simulink model "E_nonlinearB"  (R2017a)
settings: Solver=FixedStepAuto  StartTime=0.0  StopTime=200  FixedStep=sim_time  RelTol=1e-3  EnableMultiTasking=on
values from neighbouring files (symbols this model uses):
  B = [1 0.5 -0.5 -1 0 0.5 ; 0 0 0 0 2 0 ; -0.05 -0.02 0.02 0.05 0 2 ; -1 -1 -1 -1 -2 0]    [A_runSimulation.m]    (also in C_runSimulation.m; D_runSimulation.m; E_runSimulation.m; F_runSimulation.m)
  gain_four = rand()*2    [A_runSimulation.m]    (also in C_runSimulation.m = 0; D_runSimulation.m; E_runSimulation.m = 0; F_runSimulation.m = 0)
  gain_one = rand()*2    [A_runSimulation.m]    (also in C_runSimulation.m = 0; D_runSimulation.m; E_runSimulation.m = 0; F_runSimulation.m = 0)
  gain_three = rand()*2    [A_runSimulation.m]    (also in C_runSimulation.m = 0; D_runSimulation.m; E_runSimulation.m = 0; F_runSimulation.m = 0)
  gain_two = rand()*2    [A_runSimulation.m]    (also in C_runSimulation.m = 0; D_runSimulation.m; E_runSimulation.m = 0; F_runSimulation.m = 0)
  nl_gain = j    [E_runSimulation.m]
  Ql = [0 -0.1 0 0 -0.05 0; -0.2 0 0 0 -0.1 0; 0 0 0 0.2 0.1 0; 0 0 0.1 0 0.05 0; 0 0 0 0 0 0; 0 0 0 0 0 0]    [E_runSimulation.m]
  Qm = [0 0 0 0 -0.1 0; 0 0 0 0 -0.2 0; 0 0 0 0 -0.2 0; 0 0 0 0 -0.1 0; 0 0 0 0 0 0; 0 0 0 0 0 0]    [E_runSimulation.m]
  Qn = [0 -0.025 0 0 0 0; -0.05 0 0 0 0 0; 0 0 0 0.05 0 0; 0 0 0 0.025 0 0; 0 0 0 0 0 0; 0 0 0 0 0 0]    [E_runSimulation.m]
  Qz = [0 -0.2 0 0 -0.05 0; -0.2 0 0 0 -0.1 0; 0 0 0 -0.2 -0.1 0; 0 0 -0.2 0 -0.05 0; 0 0 0 0 0 0; 0 0 0 0 0 0]    [E_runSimulation.m]
  seed_four = k + 30    [A_runSimulation.m]    (also in C_runSimulation.m; D_runSimulation.m; E_runSimulation.m; F_runSimulation.m)
  seed_one = k    [A_runSimulation.m]    (also in C_runSimulation.m; D_runSimulation.m; E_runSimulation.m; F_runSimulation.m)
  seed_three = k + 20    [A_runSimulation.m]    (also in C_runSimulation.m; D_runSimulation.m; E_runSimulation.m; F_runSimulation.m)
  seed_two = k + 10    [A_runSimulation.m]    (also in C_runSimulation.m; D_runSimulation.m; E_runSimulation.m; F_runSimulation.m)
  signal_gain = j    [A_runSimulation.m]    (also in C_runSimulation.m; D_runSimulation.m; E_runSimulation.m = 0.3; F_runSimulation.m)
  sim_time = 1    [E_runSimulation.m]    (also in F_runSimulation.m = 0.1; F_runSimulation2.m = 0.1; G_runSimulation.m = 0.001)
  simulate_envelope = 1    [A_runSimulation.m]    (also in C_runSimulation.m = 0; D_runSimulation.m; E_runSimulation.m = 0)
  u_lim = [[-0.5 -0.5 -0.5 -0.5 -0.5 -0.5]' [0.5 0.5 0.5 0.5 0.5 0.5]']    [A_runSimulation.m]    (also in C_runSimulation.m; D_runSimulation.m; E_runSimulation.m; F_runSimulation.m)
  udot_lim = [[2 2 2 2 2 2]']    [A_runSimulation.m]    (also in C_runSimulation.m; D_runSimulation.m; E_runSimulation.m; F_runSimulation.m)
  W = eye(6)    [A_runSimulation.m]    (also in C_runSimulation.m; D_runSimulation.m; E_runSimulation.m; F_runSimulation.m)
libraries: dspsrcs4 x8
settings Model: Creator=markvoskuijl  LastModifiedBy=Luca
settings DataIOCC: LimitDataPoints=on  SaveFormat=Array  SignalLoggingSaveFormat=ModelDataLogs
settings OptimizationCC: ExpressionDepthLimit=2147483647  LifeSpan=inf
settings DebuggingCC: UnderspecifiedInitializationDetection=Classic  MergeDetectMultiDrivingBlocksExec=none  SolverPrmCheckMsg=warning  FcnCallInpInsideContextMsg=warning  StateNameClashWarn=warning  SFUnexpectedBacktrackingDiag=warning  SFNoUnconditionalDefaultTransitionDiag=warning  SFExecutionAtInitializationDiag=none
settings HardwareCC: ProdBitPerPointer=32  ProdBitPerSizeT=32  ProdBitPerPtrDiffT=32  ProdLargestAtomicFloat=None  ProdIntDivRoundTo=Undefined  ProdEndianess=Unspecified  ProdWordSize=32  ProdHWDeviceType=32-bit Generic
settings ModelReferenceCC: PropagateSignalLabelsOutOfModel=off
settings GRTTargetCC: TargetLangStandard=C89/C90 (ANSI)  GeneratePreprocessorConditionals=Disable all  CombineOutputUpdateFcns=off  GRTInterface=on
settings ConfigComp: CovMetricSettings=dw  CovHtmlReporting=on  CovSaveCumulativeToWorkspaceVar=on  CovSaveSingleToWorkspaceVar=on  CovExternalEMLEnable=off

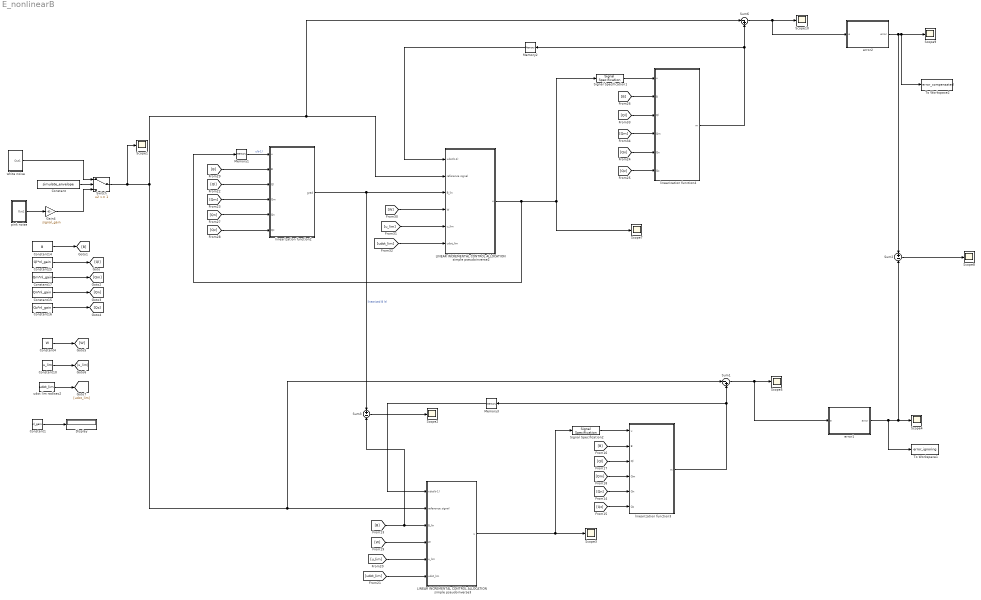
== system E_nonlinearB ==
  Constant : Constant  Value=simulate_envelope
  Constant1 : Constant  Value=nl_gain
  Constant10 : Constant  Value=u_lim
  Constant14 : Constant  Value=B
  Constant15 : Constant  Value=Qn*nl_gain
  Constant16 : Constant  Value=Qz*nl_gain
  Constant17 : Constant  Value=Qm*nl_gain
  Constant25 : Constant  Value=Ql*nl_gain
  Constant4 : Constant  Value=W
  Display : Display
  Gain4 : Gain  Gain=signal_gain
  LINEAR INCREMENTAL CONTROL ALLOCATION simple pseudoinverse2 : Subsystem
  LINEAR INCREMENTAL CONTROL ALLOCATION simple pseudoinverse3 : Subsystem
  Memory1 : Memory  X0=[0 0 0 0 0 0]
  Memory2 : Memory  X0=[0 0 0 0]
  Memory3 : Memory  X0=[0 0 0 0]
  Scope{1..5,7..10} (9 alike) : Scope
  Signal Specification1 : SignalSpecification  Dimensions=[6 1]
  Signal Specification2 : SignalSpecification  Dimensions=[6 1]
  Sum1 : Sum  Inputs=|-+
  Sum2 : Sum  Inputs=+|-
  Sum3 : Sum  Inputs=+|-
  Sum6 : Sum  Inputs=|-+
  Switch : Switch  Threshold=1
  To Workspace1 : ToWorkspace  VariableName=error_ignoring  SampleTime=-1
      settings: Save2DSignal=2-D array (concatenate along first dimension)
  To Workspace2 : ToWorkspace  VariableName=error_compensated  SampleTime=-1
      settings: Save2DSignal=2-D array (concatenate along first dimension)
  error1 : MATLAB Function  TreatAsAtomicUnit=on
  error2 : MATLAB Function  TreatAsAtomicUnit=on
  linearization function2 : MATLAB Function  TreatAsAtomicUnit=on
  linearization function3 : MATLAB Function  TreatAsAtomicUnit=on
  linearization function4 : MATLAB Function  TreatAsAtomicUnit=on
  pink noise : Subsystem
  udot lim rad/sec2 : Constant  Value=udot_lim
  white noise : Subsystem
  wires:
  Constant/1 -> Switch/2
  white noise/1(Out1) -> Switch/1
  Gain4/1 -> Switch/3
  pink noise/1(Out1) -> Gain4/1
  [W] -> LINEAR INCREMENTAL CONTROL ALLOCATION simple pseudoinverse3/4(W)
  [udot_lim] -> LINEAR INCREMENTAL CONTROL ALLOCATION simple pseudoinverse3/6(udot_lim)
  [u_lim] -> LINEAR INCREMENTAL CONTROL ALLOCATION simple pseudoinverse3/5(u_lim)
  LINEAR INCREMENTAL CONTROL ALLOCATION simple pseudoinverse3/1(u) -> Signal Specification2/1, Scope3/1
  Sum1/1 -> error1/1(e), Scope5/1
  Constant14/1 -> [B]
  Constant17/1 -> [Qm]
  Constant15/1 -> [Qn]
  Constant16/1 -> [Qz]
  Constant4/1 -> [W]
  udot lim rad/sec2/1 -> [udot_lim]
  Constant10/1 -> [u_lim]
  [B] -> linearization function3/2(B)
  [Ql] -> linearization function3/3(Ql)
  [Qn] -> linearization function3/5(Qn)
  [Qz] -> linearization function3/6(Qz)
  [Qm] -> linearization function3/4(Qm)
  error1/1(error) -> To Workspace1/1, Sum2/2, Scope4/1
  [Qz] -> linearization function2/6(Qz)
  [Ql] -> linearization function4/3(Ql)
  [B] -> linearization function4/2(B)
  [Qn] -> linearization function4/5(Qn)
  [u_lim] -> LINEAR INCREMENTAL CONTROL ALLOCATION simple pseudoinverse2/5(u_lim)
  Memory1/1 -> linearization function2/1(u)  "u(t-1)"
  Sum6/1 -> error2/1(e), Scope10/1
  linearization function2/1(grad) -> LINEAR INCREMENTAL CONTROL ALLOCATION simple pseudoinverse2/3(B_lin), Sum3/1  "linearized B (t)"
  Sum2/1 -> Scope8/1
  [udot_lim] -> LINEAR INCREMENTAL CONTROL ALLOCATION simple pseudoinverse2/6(udot_lim)
  [Ql] -> linearization function2/3(Ql)
  [W] -> LINEAR INCREMENTAL CONTROL ALLOCATION simple pseudoinverse2/4(W)
  [Qz] -> linearization function4/6(Qz)
  [Qn] -> linearization function2/5(Qn)
  [Qm] -> linearization function2/4(Qm)
  [B] -> linearization function2/2(B)
  [Qm] -> linearization function4/4(Qm)
  Memory2/1 -> LINEAR INCREMENTAL CONTROL ALLOCATION simple pseudoinverse2/1(xdot(t-1))
  Signal Specification1/1 -> linearization function4/1(u)
  Signal Specification2/1 -> linearization function3/1(u)
  Memory3/1 -> LINEAR INCREMENTAL CONTROL ALLOCATION simple pseudoinverse3/1(xdot(t-1))
  linearization function3/1(m) -> Memory3/1, Sum1/2
  Sum3/1 -> Scope2/1
  [B] -> LINEAR INCREMENTAL CONTROL ALLOCATION simple pseudoinverse3/3(B_lin), Sum3/2
  Constant25/1 -> [Ql]
  Switch/1 -> Sum6/1, LINEAR INCREMENTAL CONTROL ALLOCATION simple pseudoinverse2/2(reference signal), LINEAR INCREMENTAL CONTROL ALLOCATION simple pseudoinverse3/2(reference signal), Sum1/1, Scope1/1
  error2/1(error) -> Scope9/1, To Workspace2/1, Sum2/1
  LINEAR INCREMENTAL CONTROL ALLOCATION simple pseudoinverse2/1(u) -> Signal Specification1/1, Scope7/1, Memory1/1
  linearization function4/1(m) -> Memory2/1, Sum6/2
  Constant1/1 -> Display/1

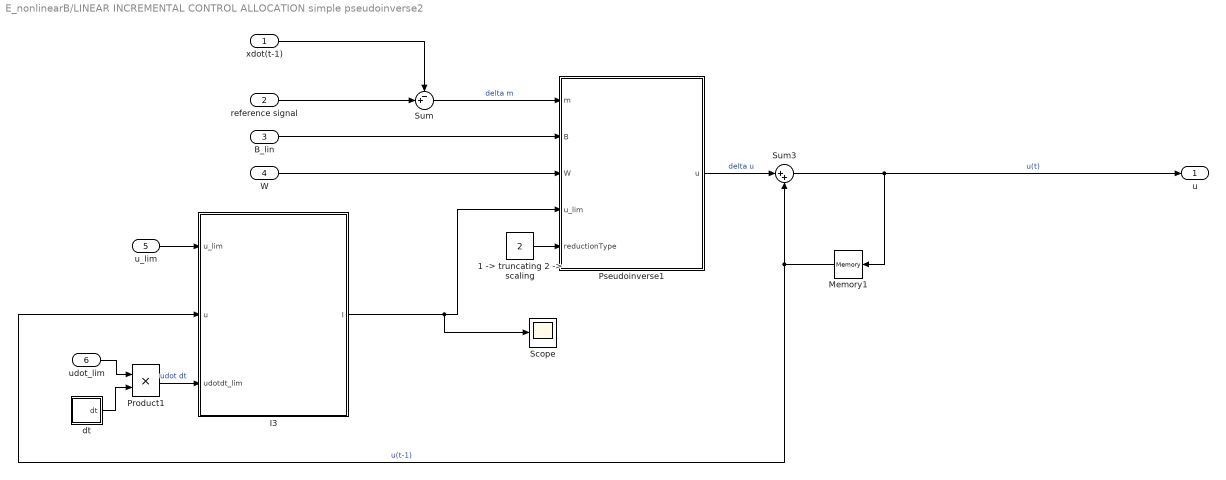
== system E_nonlinearB/LINEAR INCREMENTAL CONTROL ALLOCATION simple pseudoinverse2 ==
  xdot(t-1) : Inport
  reference signal : Inport  Port=2
  B_lin : Inport  Port=3
  W : Inport  Port=4
  u_lim : Inport  Port=5
  udot_lim : Inport  Port=6
  "1 -> truncating 2 -> scaling" : Constant  Value=2
  I3 : MATLAB Function  TreatAsAtomicUnit=on
  Memory1 : Memory
  Product1 : Product
  Pseudoinverse1 : MATLAB Function  TreatAsAtomicUnit=on
  Scope : Scope
  Sum : Sum  Inputs=-+|
  Sum3 : Sum  Inputs=|++
  dt : Subsystem
  u : Outport
  wires:
  reference signal/1 -> Sum/2
  I3/1(I) -> Scope/1, Pseudoinverse1/4(u_lim)
  Memory1/1 -> I3/2(u), Sum3/2  "u(t-1)"
  Product1/1 -> I3/3(udotdt_lim)  "udot dt"
  udot_lim/1 -> Product1/1
  Sum3/1 -> u/1, Memory1/1  "u(t)"
  Pseudoinverse1/1(u) -> Sum3/1  "delta u"
  dt/1(dt) -> Product1/2
  Sum/1 -> Pseudoinverse1/1(m)  "delta m"
  B_lin/1 -> Pseudoinverse1/2(B)
  u_lim/1 -> I3/1(u_lim)
  W/1 -> Pseudoinverse1/3(W)
  "1 -> truncating 2 -> scaling"/1 -> Pseudoinverse1/5(reductionType)
  xdot(t-1)/1 -> Sum/1

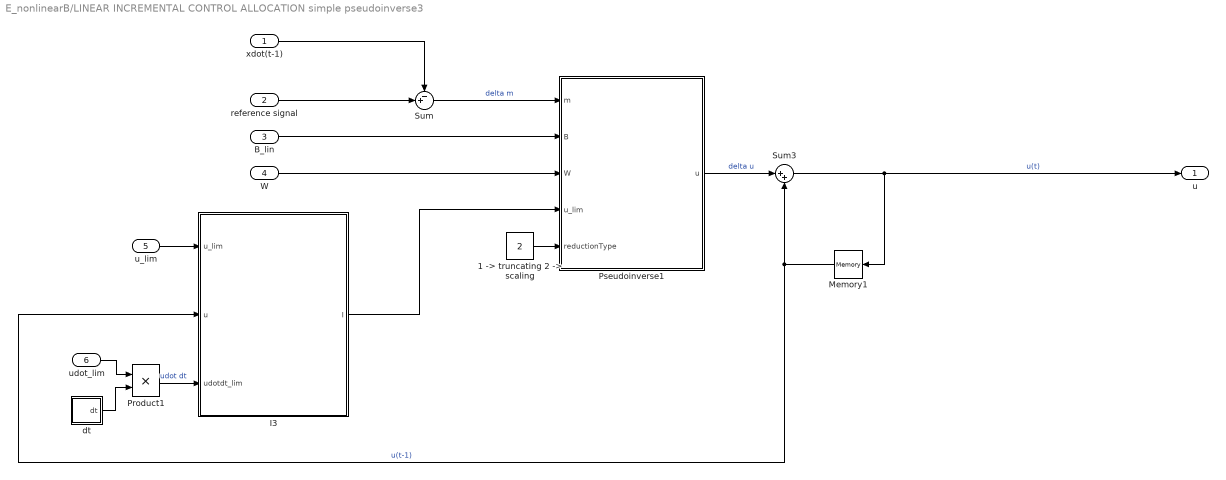
== system E_nonlinearB/LINEAR INCREMENTAL CONTROL ALLOCATION simple pseudoinverse3 ==
  xdot(t-1) : Inport
  reference signal : Inport  Port=2
  B_lin : Inport  Port=3
  W : Inport  Port=4
  u_lim : Inport  Port=5
  udot_lim : Inport  Port=6
  "1 -> truncating 2 -> scaling" : Constant  Value=2
  I3 : MATLAB Function  TreatAsAtomicUnit=on
  Memory1 : Memory
  Product1 : Product
  Pseudoinverse1 : MATLAB Function  TreatAsAtomicUnit=on
  Sum : Sum  Inputs=-+|
  Sum3 : Sum  Inputs=|++
  dt : Subsystem
  u : Outport
  wires:
  reference signal/1 -> Sum/2
  I3/1(I) -> Pseudoinverse1/4(u_lim)
  Memory1/1 -> I3/2(u), Sum3/2  "u(t-1)"
  Product1/1 -> I3/3(udotdt_lim)  "udot dt"
  udot_lim/1 -> Product1/1
  Sum3/1 -> u/1, Memory1/1  "u(t)"
  Pseudoinverse1/1(u) -> Sum3/1  "delta u"
  dt/1(dt) -> Product1/2
  Sum/1 -> Pseudoinverse1/1(m)  "delta m"
  B_lin/1 -> Pseudoinverse1/2(B)
  u_lim/1 -> I3/1(u_lim)
  W/1 -> Pseudoinverse1/3(W)
  "1 -> truncating 2 -> scaling"/1 -> Pseudoinverse1/5(reductionType)
  xdot(t-1)/1 -> Sum/1

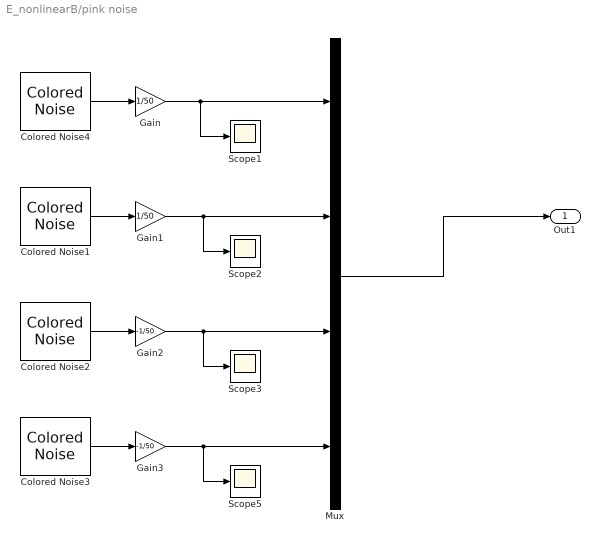
== system E_nonlinearB/pink noise ==
  Colored Noise1 : dspsrcs4/Colored Noise  Color=custom  InverseFrequencyPower=2  NumChannels=1  OutputDataType=single  SamplesPerFrame=1  SampleTime=sim_time  RandomStream=mt19937ar with seed  Seed=seed_two  SimulateUsing=Interpreted execution
      settings: SourceProductName=DSP System Toolbox  SourceProductBaseCode=DS
  Colored Noise2 : dspsrcs4/Colored Noise  Color=custom  InverseFrequencyPower=2  NumChannels=1  OutputDataType=single  SamplesPerFrame=1  SampleTime=sim_time  RandomStream=mt19937ar with seed  Seed=seed_three  SimulateUsing=Interpreted execution
      settings: SourceProductName=DSP System Toolbox  SourceProductBaseCode=DS
  Colored Noise3 : dspsrcs4/Colored Noise  Color=custom  InverseFrequencyPower=2  NumChannels=1  OutputDataType=single  SamplesPerFrame=1  SampleTime=sim_time  RandomStream=mt19937ar with seed  Seed=seed_four  SimulateUsing=Interpreted execution
      settings: SourceProductName=DSP System Toolbox  SourceProductBaseCode=DS
  Colored Noise4 : dspsrcs4/Colored Noise  Color=custom  InverseFrequencyPower=2  NumChannels=1  OutputDataType=single  SamplesPerFrame=1  SampleTime=sim_time  RandomStream=mt19937ar with seed  Seed=seed_one  SimulateUsing=Interpreted execution
      settings: SourceProductName=DSP System Toolbox  SourceProductBaseCode=DS
  Gain : Gain  Gain=1/50
  Gain1 : Gain  Gain=1/50
  Gain2 : Gain  Gain=-1/50
  Gain3 : Gain  Gain=-1/50
  Mux : Mux
  Scope{1..3,5} (4 alike) : Scope
  Out1 : Outport
  wires:
  Colored Noise4/1 -> Gain/1
  Colored Noise1/1 -> Gain1/1
  Colored Noise2/1 -> Gain2/1
  Gain/1 -> Scope1/1, Mux/1
  Gain1/1 -> Scope2/1, Mux/2
  Gain2/1 -> Scope3/1, Mux/3
  Mux/1 -> Out1/1
  Gain3/1 -> Mux/4, Scope5/1
  Colored Noise3/1 -> Gain3/1

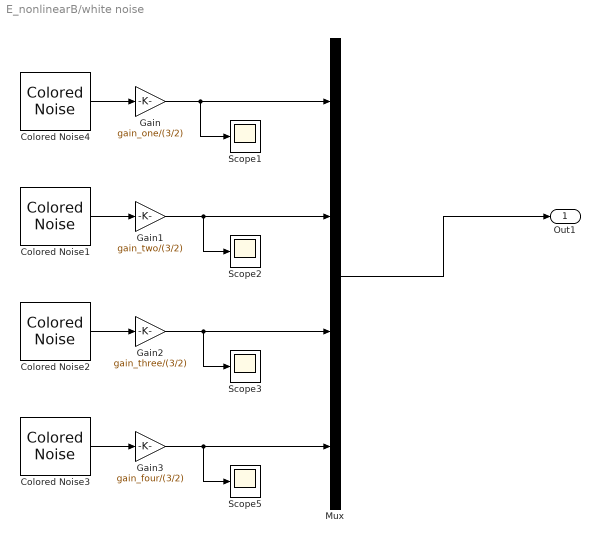
== system E_nonlinearB/white noise ==
  Colored Noise1 : dspsrcs4/Colored Noise  Color=white  InverseFrequencyPower=2  NumChannels=1  OutputDataType=single  SamplesPerFrame=1  SampleTime=sim_time  RandomStream=mt19937ar with seed  Seed=seed_two  SimulateUsing=Interpreted execution
      settings: SourceProductName=DSP System Toolbox  SourceProductBaseCode=DS
  Colored Noise2 : dspsrcs4/Colored Noise  Color=white  InverseFrequencyPower=2  NumChannels=1  OutputDataType=single  SamplesPerFrame=1  SampleTime=sim_time  RandomStream=mt19937ar with seed  Seed=seed_three  SimulateUsing=Interpreted execution
      settings: SourceProductName=DSP System Toolbox  SourceProductBaseCode=DS
  Colored Noise3 : dspsrcs4/Colored Noise  Color=white  InverseFrequencyPower=2  NumChannels=1  OutputDataType=single  SamplesPerFrame=1  SampleTime=sim_time  RandomStream=mt19937ar with seed  Seed=seed_four  SimulateUsing=Interpreted execution
      settings: SourceProductName=DSP System Toolbox  SourceProductBaseCode=DS
  Colored Noise4 : dspsrcs4/Colored Noise  Color=white  InverseFrequencyPower=2  NumChannels=1  OutputDataType=single  SamplesPerFrame=1  SampleTime=sim_time  RandomStream=mt19937ar with seed  Seed=seed_one  SimulateUsing=Interpreted execution
      settings: SourceProductName=DSP System Toolbox  SourceProductBaseCode=DS
  Gain : Gain  Gain=gain_one/(3/2)
  Gain1 : Gain  Gain=gain_two/(3/2)
  Gain2 : Gain  Gain=gain_three/(3/2)
  Gain3 : Gain  Gain=gain_four/(3/2)
  Mux : Mux
  Scope{1..3,5} (4 alike) : Scope
  Out1 : Outport
  wires:
  Colored Noise4/1 -> Gain/1
  Colored Noise1/1 -> Gain1/1
  Colored Noise2/1 -> Gain2/1
  Gain/1 -> Scope1/1, Mux/1
  Gain1/1 -> Scope2/1, Mux/2
  Gain2/1 -> Scope3/1, Mux/3
  Mux/1 -> Out1/1
  Gain3/1 -> Mux/4, Scope5/1
  Colored Noise3/1 -> Gain3/1

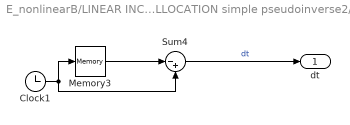
== system E_nonlinearB/LINEAR INCREMENTAL CONTROL ALLOCATION simple pseudoinverse2/dt ==
  Clock1 : Clock
  Memory3 : Memory
  Sum4 : Sum  Inputs=|-+
  dt : Outport
  wires:
  Clock1/1 -> Sum4/2, Memory3/1
  Memory3/1 -> Sum4/1
  Sum4/1 -> dt/1  "dt"

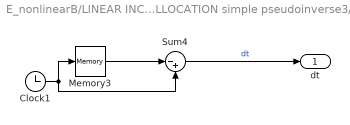
== system E_nonlinearB/LINEAR INCREMENTAL CONTROL ALLOCATION simple pseudoinverse3/dt ==
  Clock1 : Clock
  Memory3 : Memory
  Sum4 : Sum  Inputs=|-+
  dt : Outport
  wires:
  Clock1/1 -> Sum4/2, Memory3/1
  Memory3/1 -> Sum4/1
  Sum4/1 -> dt/1  "dt"

== matlab function E_nonlinearB/LINEAR INCREMENTAL CONTROL ALLOCATION simple pseudoinverse2/I3 ==
  data: u_lim input; u input; udotdt_lim input; I output
function I = computeIntersection(u_lim, u, udotdt_lim)
%check if the matrices are correct
    if not(isequal(size(u_lim,1),size(udotdt_lim,1), size(u,1)))
        error ('input matrix dimensions do not match')
    end

%declare space of intersection
    I = zeros(length(u_lim),2);
    
    I(:,1) = -min(udotdt_lim, abs(u_lim(:,1)-u));
    I(:,2) = min(+udotdt_lim, abs(u_lim(:,2)-u));
    
end

== matlab function E_nonlinearB/LINEAR INCREMENTAL CONTROL ALLOCATION simple pseudoinverse3/Pseudoinverse1 ==
  data: m input; u output; B input; W input; u_lim input; reductionType input
function u = Pseudoinverse(m, B, W, u_lim, reductionType)
coder.varsize('u_index', 'Br', 'Wr', 'u_sat');

%check if the matrices are correct
    if not(isequal(size(u_lim,1),size(B,2),size(W,1),size(W,2))...
       && isequal(length(m),size(B,1)))
        error ('input matrix dimensions do not match')
    end
    
%assign to every equation an index    
    u_index = [1:length(u_lim)].';
    
%check the type of system and then compute the pseudoinverse 1st step
    order = size(B,2)-size(B,1);

    if order > 0 %over-determined, solution that minimizes the 2norm
        u = inv(W)*B'*inv(B*inv(W)*B')*m;
    elseif order < 0 %under-determined, solution that minimizes the error
        u = inv(B'*B)*B'*m;   
    else %order = 0, sqared thus invertiBrle
        u = inv(B)*m;
    end

%deifne u_sat vector
    u_sat = zeros(length(u),1);
    
%check if the first iteration solution is correct then return    
    if not(any(u < u_lim(:,1))||any(u > u_lim(:,2)))  
        return
    end
    
%The software continues only if the solution has to be reduced
%reduce their value
    switch reductionType
        case 1 %truncation
            %takes note of which one are out of their bounds
                u_sat(u < u_lim(:,1)) = 1;
                u_sat(u > u_lim(:,2)) = 1;
                
            %trucate
                u = min(u, u_lim(:,2));
                u = max(u, u_lim(:,1));

        case 2 %scaling solution -> direction preserving
            %reduce
                a = zeros(length(u),1);

                for i = 1:length(u)
                    if u(i)>0
                       a(i) = abs(u(i)/u_lim(i,2));
                    elseif u(i)<0
                       a(i) = abs(u(i)/u_lim(i,1));
                    else
                       a(i) = 0; 
                    end          
                end
                a_max = max(a);
                u = u/a_max;
            
            %takes note of which one are out of their bounds
                u_sat(u == u_lim(:,2)) = 1;
                u_sat(u == u_lim(:,1)) = 1;
            
    end
    
return
    
end

== matlab function E_nonlinearB/LINEAR INCREMENTAL CONTROL ALLOCATION simple pseudoinverse3/I3 ==
  data: u_lim input; u input; udotdt_lim input; I output
function I = computeIntersection(u_lim, u, udotdt_lim)
%check if the matrices are correct
    if not(isequal(size(u_lim,1),size(udotdt_lim,1), size(u,1)))
        error ('input matrix dimensions do not match')
    end

%declare space of intersection
    I = zeros(length(u_lim),2);
    
    I(:,1) = -min(udotdt_lim, abs(u_lim(:,1)-u));
    I(:,2) = min(+udotdt_lim, abs(u_lim(:,2)-u));
    
end

== matlab function E_nonlinearB/linearization function3 ==
  data: u input; B input; m output; Ql input; Qm input; Qn input; Qz input
function m = moment(u, B, Ql, Qm, Qn, Qz)
%the equation here implemented comes from the article
%"A method fot including control effector interactions in the control
%allocation problem" by Oppenheimer but it is addressed to control also z
%The equation is posed in te form:

%             |u' Ql|
%             |u' Qm|
%   g = 1/2 * |u' Qn| + B
%             |u' Qz|

m = ((1/2)*([u.'*Ql; u.'*Qm; u.'*Qn; u.'*Qz])+B)*u;

end

== matlab function E_nonlinearB/error1 ==
  data: e input; error output
function error = error(e)

    error = sum(abs(e));

end

== matlab function E_nonlinearB/LINEAR INCREMENTAL CONTROL ALLOCATION simple pseudoinverse2/Pseudoinverse1 ==
  data: m input; u output; B input; W input; u_lim input; reductionType input
function u = Pseudoinverse(m, B, W, u_lim, reductionType)
coder.varsize('u_index', 'Br', 'Wr', 'u_sat');

%check if the matrices are correct
    if not(isequal(size(u_lim,1),size(B,2),size(W,1),size(W,2))...
       && isequal(length(m),size(B,1)))
        error ('input matrix dimensions do not match')
    end
    
%assign to every equation an index    
    u_index = [1:length(u_lim)].';
    
%check the type of system and then compute the pseudoinverse 1st step
    order = size(B,2)-size(B,1);

    if order > 0 %over-determined, solution that minimizes the 2norm
        u = inv(W)*B'*inv(B*inv(W)*B')*m;
    elseif order < 0 %under-determined, solution that minimizes the error
        u = inv(B'*B)*B'*m;   
    else %order = 0, sqared thus invertiBrle
        u = inv(B)*m;
    end

%deifne u_sat vector
    u_sat = zeros(length(u),1);
    
%check if the first iteration solution is correct then return    
    if not(any(u < u_lim(:,1))||any(u > u_lim(:,2)))  
        return
    end
    
%The software continues only if the solution has to be reduced
%reduce their value
    switch reductionType
        case 1 %truncation
            %takes note of which one are out of their bounds
                u_sat(u < u_lim(:,1)) = 1;
                u_sat(u > u_lim(:,2)) = 1;
                
            %trucate
                u = min(u, u_lim(:,2));
                u = max(u, u_lim(:,1));

        case 2 %scaling solution -> direction preserving
            %reduce
                a = zeros(length(u),1);

                for i = 1:length(u)
                    if u(i)>0
                       a(i) = abs(u(i)/u_lim(i,2));
                    elseif u(i)<0
                       a(i) = abs(u(i)/u_lim(i,1));
                    else
                       a(i) = 0; 
                    end          
                end
                a_max = max(a);
                u = u/a_max;
            
            %takes note of which one are out of their bounds
                u_sat(u == u_lim(:,2)) = 1;
                u_sat(u == u_lim(:,1)) = 1;
            
    end
    
    u = real(u);
return
    
end

== matlab function E_nonlinearB/error2 ==
  data: e input; error output
function error = error(e)

    error = sum(abs(e));

end

== matlab function E_nonlinearB/linearization function2 ==
  data: u input; B input; grad output; Ql input; Qm input; Qn input; Qz input
function grad = linearizeSystem(u, B, Ql, Qm, Qn, Qz)
%the equation here implemented comes from the article
%"A method fot including control effector interactions in the control
%allocation problem" by Oppenheimer but it is addressed to control also z
%The equation is posed in te form:

%             |u' Ql|
%             |u' Qm|
%   g = 1/2 * |u' Qn| + B
%             |u' Qz|

%and must be linearized into a new control effectiveness matrix



%check the magnitude of numbers inside the matrices
%     oom = [min(floor(log10(u+1))), min(min(floor(log10(Ql+1)))),...
%         min(min(floor(log10(Qm+1)))), min(min(floor(log10(Qn+1)))),...
%         min(min(floor(log10(Qz+1))))];
%     oom = min(oom);

oom = -1;
 
%compute the gradient that will be the new B matrix
    grad = zeros(size(B,1),length(u));
    
    ddelta = 10^(oom-5); %three orders of magnitude less than the values in the matrices
    for i = 1:length(u)
        u_base = u;
        u_incr = u; u_incr(i) = u_incr(i)+ddelta;
        u_decr = u; u_decr(i) = u_decr(i)-ddelta;
        
        g_base = ((1/2)*([u_base.'*Ql; u_base.'*Qm; u_base.'*Qn; u_base.'*Qz])+B)*u_base;
        g_incr = ((1/2)*([u_incr.'*Ql; u_incr.'*Qm; u_incr.'*Qn; u_incr.'*Qz])+B)*u_incr;
        g_decr = ((1/2)*([u_decr.'*Ql; u_decr.'*Qm; u_decr.'*Qn; u_decr.'*Qz])+B)*u_decr;
        
        grad_incr = (g_incr - g_base)/ddelta;
        grad_decr = (g_decr - g_base)/(-ddelta); 
        grad(:,i) = (grad_incr+grad_decr)/2;
    end
end

== matlab function E_nonlinearB/linearization function4 ==
  data: u input; B input; m output; Ql input; Qm input; Qn input; Qz input
function m = moment(u, B, Ql, Qm, Qn, Qz)
%the equation here implemented comes from the article
%"A method fot including control effector interactions in the control
%allocation problem" by Oppenheimer but it is addressed to control also z
%The equation is posed in te form:

%             |u' Ql|
%             |u' Qm|
%   g = 1/2 * |u' Qn| + B
%             |u' Qz|

m = ((1/2)*([u.'*Ql; u.'*Qm; u.'*Qn; u.'*Qz])+B)*u;
m = real(m);
end
